simulink model "L_PLL"  (R2021a)
settings: Solver=VariableStepAuto  StartTime=0.0  StopTime=2  RelTol=1e-3
undefined symbols (not defined in the file or in its folder): DiscIntNeverNeededParam, i
libraries: spsACVoltageSourceLib x2, spsVoltageMeasurementLib x2, dspsigops x2, spsAlphaBetaZerotodq0Lib x1, simulink x1, spspowerguiLib x1
settings Model: Creator=negis  LastModifiedBy=negis

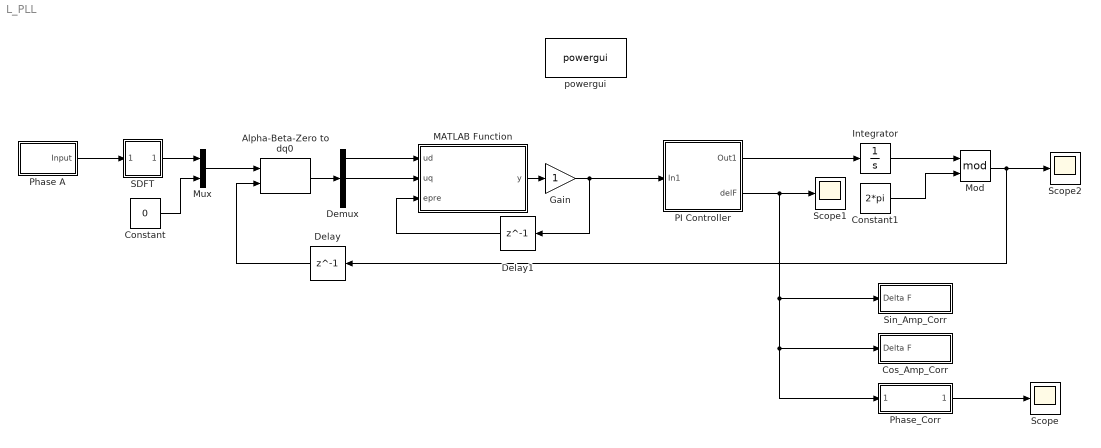
== system L_PLL ==
  Alpha-Beta-Zero to dq0 : spsAlphaBetaZerotodq0Lib/Alpha-Beta-Zero to dq0  Alignment=90 degrees behind phase A axis
      settings: SourceProductBaseCode=PS
  Constant : Constant  Value=0
  Constant1 : Constant  Value=2*pi
  Cos_Amp_Corr : Subsystem
  Delay : Delay  DelayLength=1  InitialCondition=0
  Delay1 : Delay  DelayLength=1  InitialCondition=0
  Demux : Demux  Outputs=3
  Gain : Gain
  Integrator : Integrator
  MATLAB Function : MATLAB Function  TreatAsAtomicUnit=on
  Mod : Math  Operator=mod  SignedPower=on  SaturateOnIntegerOverflow=on
  Mux : Mux  Inputs=2
  PI Controller : Subsystem
  Phase A : Subsystem
  Phase_Corr : Subsystem
  SDFT : Subsystem
  Scope : Scope
  Scope1 : Scope
  Scope2 : Scope
  Sin_Amp_Corr : Subsystem
  powergui : spspowerguiLib/powergui  Priority=1  SimulationMode=Discrete  SampleTime=50e-6  frequency=60  Iterations=50  frequencyindice=50  Pbase=100e6  ErrMax=1e-4  UnitsV=kV  UnitsW=MW  buscounter=0  FunctionMessages=off  echomessages=off  EnableUseOfTLC=off  CurrentSourceSwitches=off  DisableSnubberDevices=off  DisableRonSwitches=off  DisableVfSwitches=off  DisplayEquations=off  AutomaticDiscreteSolvers=off  SolverType=Tustin/Backward Euler (TBE)  Interpol=off  ExternalGateDelay=off  methode=off  Ts=100  x0status=blocks  SPID=on  SwTol=0  HookPort=off  NonlinearTolerance=1e-4  nMaxIteration=100  ContinueOnMaxIteration=off  RestoreLinks=warning  ResistiveCurrentMeasurement=off  Frange=[0:2:500]  Ylog=off  Xlog=on  ShowGrid=off  save=off  variable=ZData  structure=0  ZoomFFT=off  StartTime=0.0  cycles=1  DisplayStyle=1  fundamental=60  FreqAxis=off  MaxFrequency=1000  frequencyindicesteady=1  RmsSteady=1  display=off
  wires:
  Delay1/1 -> MATLAB Function/3(epre)
  Gain/1 -> PI Controller/1(In1), Delay1/1
  Constant/1 -> Mux/2
  Delay/1 -> Alpha-Beta-Zero to dq0/2
  Phase_Corr/1(Outport) -> Scope/1
  Integrator/1 -> Mod/1
  PI Controller/2(delF) -> Scope1/1, Sin_Amp_Corr/1(Delta F), Cos_Amp_Corr/1(Delta F), Phase_Corr/1(Delta F)
  Demux/2 -> MATLAB Function/2(uq)
  Mux/1 -> Alpha-Beta-Zero to dq0/1
  Constant1/1 -> Mod/2
  Alpha-Beta-Zero to dq0/1 -> Demux/1
  MATLAB Function/1(y) -> Gain/1
  Mod/1 -> Scope2/1, Delay/1
  PI Controller/1(Out1) -> Integrator/1
  Demux/1 -> MATLAB Function/1(ud)
  SDFT/1(Out) -> Mux/1
  Phase A/1(Input) -> SDFT/1(Input)

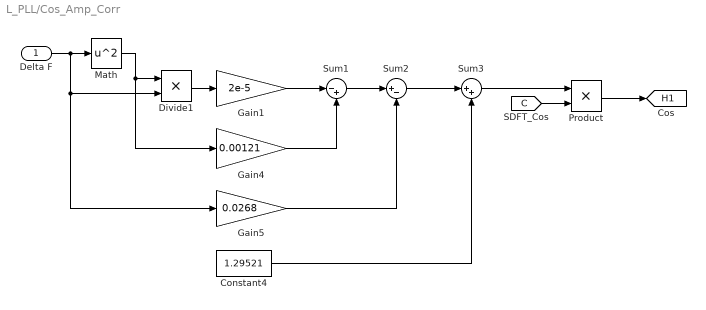
== system L_PLL/Cos_Amp_Corr ==
  Delta F : Inport
  Constant4 : Constant  Value=1.29521
  Divide1 : Product  Inputs=**
  Gain1 : Gain  Gain=2e-5  RndMeth=Nearest
  Gain4 : Gain  Gain=0.00121  RndMeth=Nearest
  Gain5 : Gain  Gain=0.0268
  "Math " : Math  Operator=square  SignedPower=on  SaturateOnIntegerOverflow=on
  Product : Product
  Sum1 : Sum  Inputs=|-+  RndMeth=Nearest
  Sum2 : Sum  Inputs=|+-  RndMeth=Nearest
  Sum3 : Sum  Inputs=|++  RndMeth=Nearest
  tag scope: H1=global
  wires:
  Delta F/1 -> "Math "/1, Divide1/2, Gain5/1
  "Math "/1 -> Divide1/1, Gain4/1
  Divide1/1 -> Gain1/1
  Gain1/1 -> Sum1/1
  Gain4/1 -> Sum1/2
  Gain5/1 -> Sum2/2
  Sum1/1 -> Sum2/1
  Sum2/1 -> Sum3/1
  Constant4/1 -> Sum3/2
  Product/1 -> [H1]
  Sum3/1 -> Product/1
  [C] -> Product/2

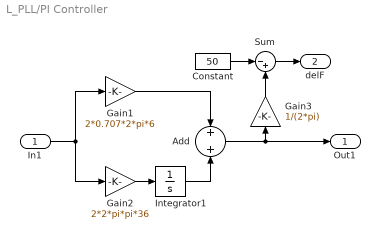
== system L_PLL/PI Controller ==
  In1 : Inport
  Add : Sum
  Constant : Constant  Value=50
  Gain1 : Gain  Gain=2*0.707*2*pi*6
  Gain2 : Gain  Gain=2*2*pi*pi*36
  Gain3 : Gain  Gain=1/(2*pi)
  Integrator1 : Integrator
  Sum : Sum  Inputs=|-+
  Out1 : Outport
  delF : Outport  Port=2
  wires:
  Gain1/1 -> Add/1
  Integrator1/1 -> Add/2
  In1/1 -> Gain1/1, Gain2/1
  Gain2/1 -> Integrator1/1
  Add/1 -> Out1/1, Gain3/1
  Sum/1 -> delF/1
  Constant/1 -> Sum/1
  Gain3/1 -> Sum/2

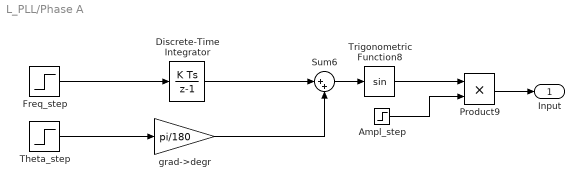
== system L_PLL/Phase A ==
  Ampl_step : Step  Before=230*sqrt(2)  After=230*sqrt(2)  SampleTime=0.0001
  Discrete-Time Integrator : DiscreteIntegrator  SampleTime=-1  ICPrevOutput=DiscIntNeverNeededParam  ICPrevScaledInput=DiscIntNeverNeededParam
  Freq_step : Step  Before=2*pi*50  After=2*pi*50  SampleTime=0.0001  VectorParams1D=off
  Product9 : Product  RndMeth=Zero
  Sum6 : Sum  Inputs=|++  InputSameDT=on  SaturateOnIntegerOverflow=on  OutDataTypeStr=Inherit: Same as first input
  Theta_step : Step  After=0  SampleTime=0.0001
  Trigonometric Function8 : Trigonometry
  grad->degr : Gain  Gain=pi/180  SaturateOnIntegerOverflow=on  OutDataTypeStr=Inherit: Same as input  ParamDataTypeStr=Inherit: Same as input
  Input : Outport
  wires:
  grad->degr/1 -> Sum6/2
  Ampl_step/1 -> Product9/2
  Sum6/1 -> Trigonometric Function8/1
  Freq_step/1 -> Discrete-Time Integrator/1
  Trigonometric Function8/1 -> Product9/1
  Product9/1 -> Input/1
  Discrete-Time Integrator/1 -> Sum6/1
  Theta_step/1 -> grad->degr/1

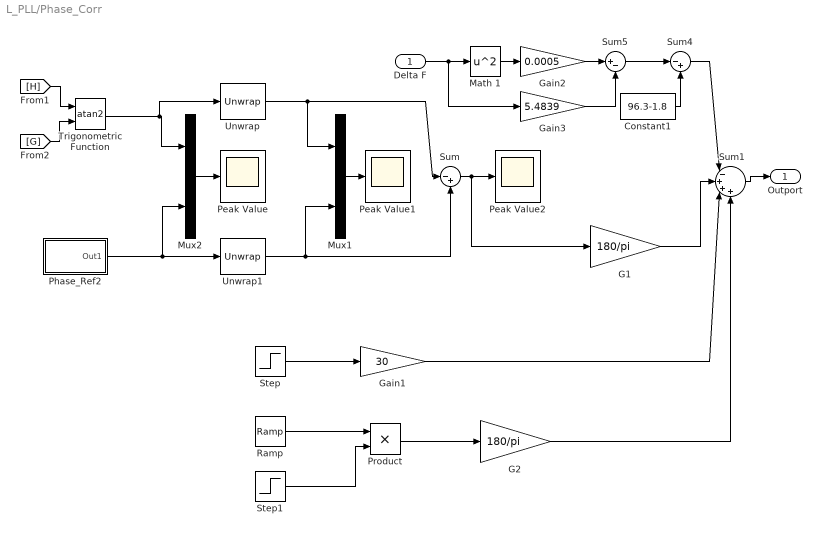
== system L_PLL/Phase_Corr ==
  Delta F : Inport
  Constant1 : Constant  Value=96.3-1.8
  G1 : Gain  Gain=180/pi
  G2 : Gain  Gain=180/pi
  Gain1 : Gain  Gain=30  RndMeth=Nearest
  Gain2 : Gain  Gain=0.0005  RndMeth=Nearest
  Gain3 : Gain  Gain=5.4839
  Math 1 : Math  Operator=square  SignedPower=on  SaturateOnIntegerOverflow=on
  Mux1 : Mux  Inputs=2
  Mux2 : Mux  Inputs=2
  Peak Value : Scope
  Peak Value1 : Scope
  Peak Value2 : Scope
  Phase_Ref2 : Subsystem
  Product : Product
  Ramp : simulink/Sources/Ramp  slope=2*pi*1  start=0.65  InitialOutput=0
  Step : Step  Time=0.65  SampleTime=1/(10000)
  Step1 : Step  Time=0.65  SampleTime=1/10000
  Sum : Sum  Inputs=|-+
  Sum1 : Sum  Inputs=|-+++
  Sum4 : Sum  Inputs=|-+  RndMeth=Nearest
  Sum5 : Sum  Inputs=|+-  RndMeth=Nearest
  Trigonometric Function : Trigonometry  Operator=atan2
  Unwrap : dspsigops/Unwrap  tol=pi/2  running=off
  Unwrap1 : dspsigops/Unwrap  tol=pi/2  running=off
  Outport : Outport
  wires:
  [G] -> Trigonometric Function/2
  [H] -> Trigonometric Function/1
  Trigonometric Function/1 -> Unwrap/1, Mux2/1
  Mux2/1 -> Peak Value/1
  Mux1/1 -> Peak Value1/1
  Unwrap/1 -> Sum/1, Mux1/1
  Unwrap1/1 -> Sum/2, Mux1/2
  Sum/1 -> G1/1, Peak Value2/1
  Phase_Ref2/1(Out1) -> Mux2/2, Unwrap1/1
  G1/1 -> Sum1/2
  Constant1/1 -> Sum4/2
  Gain3/1 -> Sum5/2
  Gain2/1 -> Sum5/1
  Delta F/1 -> Gain3/1, Math 1/1
  Math 1/1 -> Gain2/1
  Sum5/1 -> Sum4/1
  Sum4/1 -> Sum1/1
  Sum1/1 -> Outport/1
  Step/1 -> Gain1/1
  Ramp/1 -> Product/1
  Step1/1 -> Product/2
  Product/1 -> G2/1
  G2/1 -> Sum1/4
  Gain1/1 -> Sum1/3

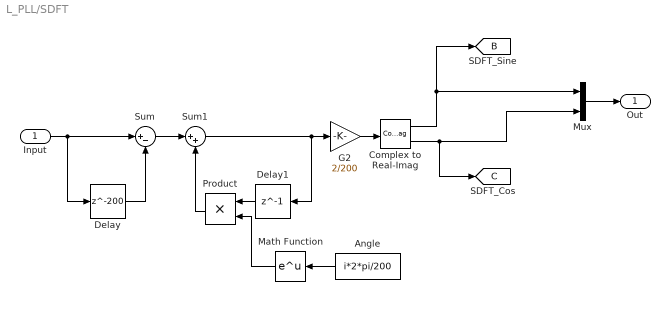
== system L_PLL/SDFT ==
  Input : Inport
  Angle : Constant  Value=i*2*pi/200
  Complex to Real-Imag : ComplexToRealImag
  Delay : Delay  DelayLength=200  InitialCondition=0
  Delay1 : Delay  DelayLength=1  InitialCondition=0
  G2 : Gain  Gain=2/200
  Math Function : Math  SignedPower=on  SaturateOnIntegerOverflow=on
  Mux : Mux  Inputs=2
  Product : Product
  Sum : Sum  Inputs=|+-
  Sum1 : Sum  Inputs=|++
  Out : Outport
  tag scope: B=global, C=global
  wires:
  Delay/1 -> Sum/2
  Sum/1 -> Sum1/1
  Sum1/1 -> G2/1, Delay1/1
  Delay1/1 -> Product/1
  Product/1 -> Sum1/2
  Complex to Real-Imag/2 -> Mux/2, [C]
  Angle/1 -> Math Function/1
  G2/1 -> Complex to Real-Imag/1
  Complex to Real-Imag/1 -> [B], Mux/1
  Math Function/1 -> Product/2
  Input/1 -> Delay/1, Sum/1
  Mux/1 -> Out/1

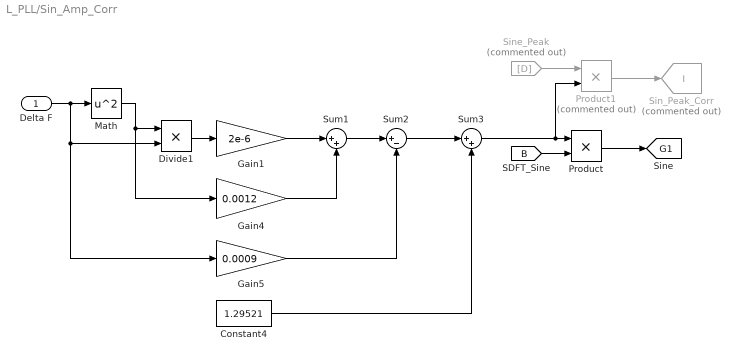
== system L_PLL/Sin_Amp_Corr ==
  Delta F : Inport
  Constant4 : Constant  Value=1.29521
  Divide1 : Product  Inputs=**
  Gain1 : Gain  Gain=2e-6  RndMeth=Nearest
  Gain4 : Gain  Gain=0.0012  RndMeth=Nearest
  Gain5 : Gain  Gain=0.0009
  "Math " : Math  Operator=square  SignedPower=on  SaturateOnIntegerOverflow=on
  Product : Product
  Product1 : Product  Commented=on
  Sin_Peak_Corr : Goto  Commented=on  GotoTag=I  TagVisibility=global
  Sine_Peak : From  Commented=on  GotoTag=D  TagVisibility=global
  Sum1 : Sum  Inputs=|++  RndMeth=Nearest
  Sum2 : Sum  Inputs=|+-  RndMeth=Nearest
  Sum3 : Sum  Inputs=|++  RndMeth=Nearest
  tag scope: G1=global
  wires:
  Delta F/1 -> "Math "/1, Divide1/2, Gain5/1
  "Math "/1 -> Divide1/1, Gain4/1
  Divide1/1 -> Gain1/1
  Gain1/1 -> Sum1/1
  Gain4/1 -> Sum1/2
  Gain5/1 -> Sum2/2
  Sum1/1 -> Sum2/1
  Sum2/1 -> Sum3/1
  Constant4/1 -> Sum3/2
  Product/1 -> [G1]
  Sum3/1 -> Product1/2, Product/1
  [B] -> Product/2
  Sine_Peak/1 -> Product1/1
  Product1/1 -> Sin_Peak_Corr/1

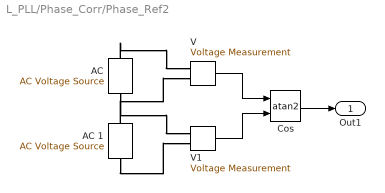
== system L_PLL/Phase_Corr/Phase_Ref2 ==
  "AC " : spsACVoltageSourceLib/AC Voltage Source  Amplitude=1  Phase=270  Frequency=50  SampleTime=0.0001  Measurements=None  BusType=swing  Pref=10e3  Qref=0  Qmin=-inf  Qmax=+inf
  AC 1 : spsACVoltageSourceLib/AC Voltage Source  Amplitude=1  Phase=0  Frequency=50  SampleTime=0.0001  Measurements=None  BusType=swing  Pref=10e3  Qref=0  Qmin=-inf  Qmax=+inf
  Cos : Trigonometry  Operator=atan2  NumberOfIterations=20
  V : spsVoltageMeasurementLib/Voltage Measurement  PhasorSimulation=off  OutputType=Complex  PSBequivalent=0
  V1 : spsVoltageMeasurementLib/Voltage Measurement  PhasorSimulation=off  OutputType=Complex  PSBequivalent=0
  Out1 : Outport
  wires:
  V/1 -> Cos/1
  V1/1 -> Cos/2
  Cos/1 -> Out1/1
  connections:
  AC 1/LConn1 -- V1/LConn2
  "AC "/LConn1 -- V/LConn2
  "AC "/RConn1 -- V/LConn1
  AC 1/RConn1 -- V1/LConn1

== matlab function L_PLL/MATLAB Function ==
  data: ud input; uq input; y output; epre input
function y = Error_Unwrap(ud,uq,epre)
zone=0;
e=atan2(uq,ud);
error = e+(2*pi*zone)-epre; 
if(error<-pi)
    zone=zone+1;
end
if(error>pi)
    zone=zone-1;
end
e = e+(2*pi*zone);
epre=e;
y = epre;
